simulink model "mount_2_rust"  (R2022b)
settings: Solver=FixedStepDiscrete  StartTime=0.0  StopTime=5  FixedStep=deltaT  RelTol=1e-3
InitFcn:
  | %
  | % Initialization callback function
  | %
  | 
  | try
  |    % fprintf('\n Simulink control model!\n');
  | 
  |    % Get Simulink model directory
  |    [filepath,name,ext] = fileparts(which(bdroot));
  | 
  |    if ~strcmp(filepath,pwd)
  |       fprintf('\n Changing current directory to \n %s \n',filepath);
  |       cd(filepath);
  |    end
  | 
  | catch
  |    warning('Running the InitFcn from puSimulate script');
  | end
values from neighbouring files (symbols this model uses):
  drv_delay = ceil(mount.delay/FEM_Ts)    [load_mount_data.m]
  FEM_Ts = deltaT    (= 0.000125)    [load_mount_data.m]
  Hdrive_d = c2d(o.Hdrive(1,1), FEM_Ts, 'tustin')    [load_mount_data.m]
  mnt_TF_Ts = FEM_Ts    (= 0.000125)    [load_mount_data.m]
  o = fun_confBase(oTest)    [load_mount_data.m]
undefined symbols (not defined in the file or in its folder): a, az, az_ff_en, b, c, DiscIntNeverNeededParam, el, gir, magnitude, mount
libraries: simulink x2, simulink_extras x2
(part 1 of 2)
settings Model: SimulationMode=accelerator  Creator=RRomano  LastModifiedBy=rromano
settings SolverCC: AlgebraicLoopSolver=TrustRegion
settings DataIOCC: SaveOutput=off  SignalLogging=off  DSMLogging=off  SaveTime=off  ReturnWorkspaceOutputs=off
settings OptimizationCC: DefaultParameterBehavior=Inlined  GainParamInheritBuiltInType=on  UseFloatMulNetSlope=on  UseSpecifiedMinMax=on  InlineInvariantSignals=on  StrengthReduction=on  PassReuseOutputArgsAs=Individual arguments  ZeroExternalMemoryAtStartup=off  ZeroInternalMemoryAtStartup=off  NoFixptDivByZeroProtection=on  EfficientFloat2IntCast=on  LifeSpan=1000  SimCompilerOptimization=on  AccelVerboseBuild=on  OptimizeBlockOrder=speed  OptimizationPriority=Speed  OptimizationCustomize=off  MultiThreadedLoops=on  EfficientTunableParamExpr=on
settings DebuggingCC: InheritedTsInSrcMsg=none  MultiTaskRateTransMsg=warning  ParameterTunabilityLossMsg=error  UnconnectedInputMsg=warning  UnconnectedOutputMsg=warning  UnconnectedLineMsg=warning  SFUnexpectedBacktrackingDiag=warning  SFNoUnconditionalDefaultTransitionDiag=warning  SFExecutionAtInitializationDiag=none  SFMachineParentedDataDiag=warning  ArithmeticOperatorsInVariantConditions=warning
settings HardwareCC: ProdBitPerLong=64  ProdLongLongMode=on  ProdHWDeviceType=Intel->x86-64 (Linux 64)  TargetBitPerLong=64  TargetBitPerPointer=64  TargetBitPerSizeT=64  TargetBitPerPtrDiffT=64  TargetLongLongMode=on  TargetIntDivRoundTo=Zero  TargetEndianess=LittleEndian  TargetWordSize=64  TargetHWDeviceType=MATLAB Host  ProdEqTarget=off
settings ModelReferenceCC: EnableRefExpFcnMdlSchedulingChecks=on
settings SFSimCC: SimUseLocalCustomCode=off  MATLABDynamicMemAlloc=off  CustomCodeUndefinedFunction=UseInterfaceOnly
settings RTWCC: Description=Embedded Coder  SystemTargetFile=ert.tlc  GenCodeOnly=on  GenerateMakefile=off  TemplateMakefile=ert_default_tmf  GenerateReport=on  BuildConfiguration=Faster Runs  RTWCompilerOptimization=on  CheckMdlBeforeBuild=Warning  DLArmComputeVersion=19.05
settings CodeAppCC: ForceParamTrailComments=on  IgnoreCustomStorageClasses=off  OperatorAnnotations=on  SimulinkDataObjDesc=on  SFDataObjDesc=on  InsertBlockDesc=on
settings ERTTargetCC: TargetLangStandard=C99 (ISO)  GenerateSampleERTMain=on  CombineSignalStateStructs=on  SuppressErrorStatus=on  CodeInterfacePackaging=Reusable function  SupportNonFinite=off  SupportComplex=off  InlinedParameterPlacement=NonHierarchical  RootIOFormat=Structure reference  ERTCustomFileTemplate=example_file_process.tlc
settings ConfigComp: CovMetricSettings=dw  CovSaveCumulativeToWorkspaceVar=on  CovSaveSingleToWorkspaceVar=on  CovExternalEMLEnable=off

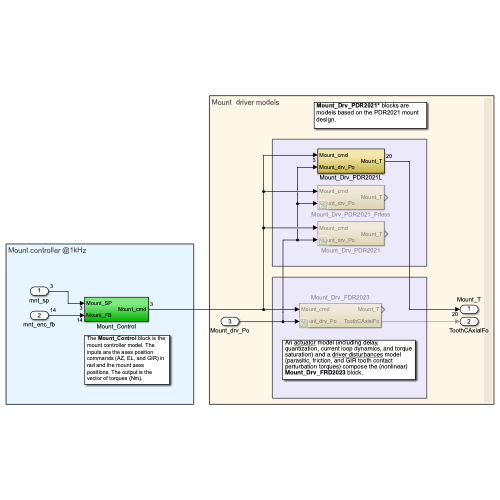
[thumbnail: Simulink's stored preview of the top-level diagram]
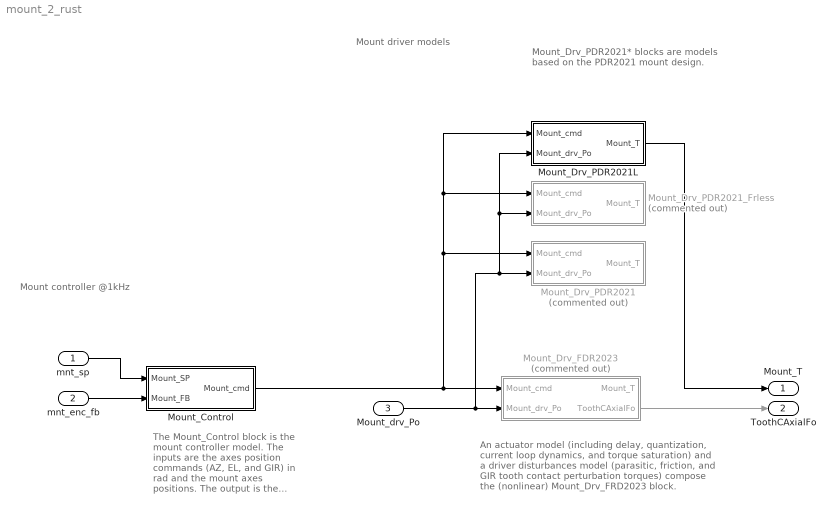
== system mount_2_rust ==
  note: Mount controller @1kHz
  note: Mount driver models
  note: The Mount_Control block is the mount controller model. The inputs are the axes position commands (AZ, EL, and GIR) in rad and the mount axes positions. The output is the vector of torques (Nm).
  note: An actuator model (including delay, quantization, current loop dynamics, and torque saturation) and a driver disturbances model (parasitic, friction, and GIR tooth contact perturbation torques) compose the (nonlinear) Mount_Drv_FRD2023 block.
  note: Mount_Drv_PDR2021* blocks are models based on the PDR2021 mount design.
  mnt_sp : Inport  SampleTime=mnt_TF_Ts
  mnt_enc_fb : Inport  Port=2  SampleTime=mnt_TF_Ts
  Mount_drv_Po : Inport  Port=3  SampleTime=FEM_Ts
  Mount_Control : Subsystem
  Mount_Drv_FDR2023 : Subsystem  Commented=on
  Mount_Drv_PDR2021 : Subsystem  Commented=on
  Mount_Drv_PDR2021L : Subsystem
  Mount_Drv_PDR2021_Frless : Subsystem  Commented=on
  Mount_T : Outport  SampleTime=FEM_Ts  VectorParamsAs1DForOutWhenUnconnected=off
  ToothCAxialFo : Outport  Port=2  SampleTime=FEM_Ts  VectorParamsAs1DForOutWhenUnconnected=off
  wires:
  mnt_sp/1 -> Mount_Control/1(Mount_SP)
  Mount_Drv_FDR2023/2(ToothCAxialFo) -> ToothCAxialFo/1
  mnt_enc_fb/1 -> Mount_Control/2(Mount_FB)
  Mount_Control/1(Mount_cmd) -> Mount_Drv_PDR2021/1(Mount_cmd), Mount_Drv_PDR2021_Frless/1(Mount_cmd), Mount_Drv_PDR2021L/1(Mount_cmd), Mount_Drv_FDR2023/1(Mount_cmd)
  Mount_drv_Po/1 -> Mount_Drv_PDR2021L/2(Mount_drv_Po), Mount_Drv_PDR2021_Frless/2(Mount_drv_Po), Mount_Drv_PDR2021/2(Mount_drv_Po), Mount_Drv_FDR2023/2(Mount_drv_Po)
  Mount_Drv_PDR2021L/1(Mount_T) -> Mount_T/1

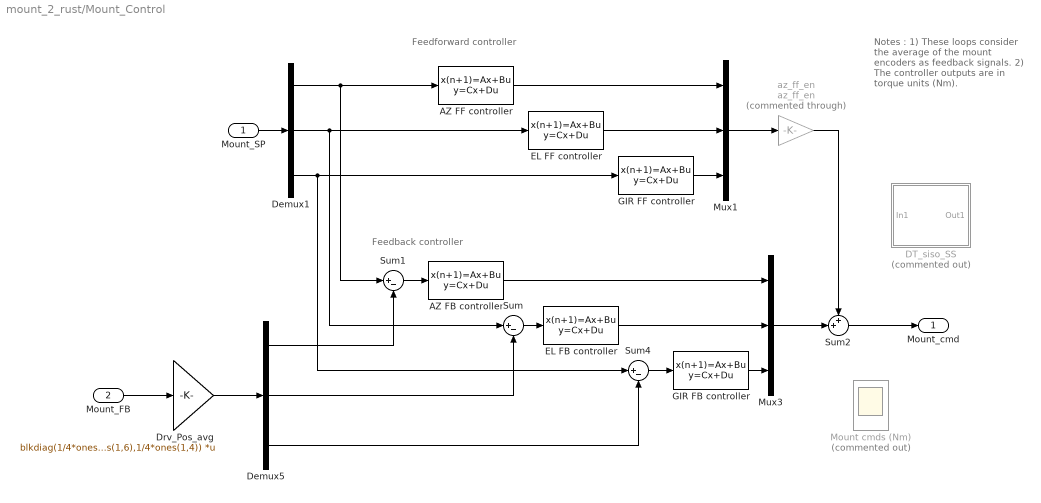
== system mount_2_rust/Mount_Control ==
  note: Feedback controller
  note: Feedforward controller
  note: Notes :
      | 1) These loops consider the average of the mount encoders as feedback signals.
      | 2) The controller outputs are in torque units (Nm).
  Mount_SP : Inport
  Mount_FB : Inport  Port=2
  AZ FB controller : DiscreteStateSpace  A=mount.az.SSdtHfb.A  B=mount.az.SSdtHfb.B  C=mount.az.SSdtHfb.C  D=mount.az.SSdtHfb.D  SampleTime=mount.az.SSdtHfb.Ts
  AZ FF controller : DiscreteStateSpace  A=mount.az.SSdtHff.A  B=mount.az.SSdtHff.B  C=mount.az.SSdtHff.C  D=mount.az.SSdtHff.D  SampleTime=mount.az.SSdtHff.Ts
  DT_siso_SS : Subsystem  Commented=on
  Demux1 : Demux  Outputs=[1,1,1]
  Demux5 : Demux  Outputs=3
  Drv_Pos_avg : Gain  Gain=blkdiag(1/4*ones(1,4),1/6*ones(1,6),1/4*ones(1,4))  Multiplication=Matrix(K*u) (u vector)
  EL FB controller : DiscreteStateSpace  A=mount.el.SSdtHfb.A  B=mount.el.SSdtHfb.B  C=mount.el.SSdtHfb.C  D=mount.el.SSdtHfb.D  SampleTime=mount.el.SSdtHfb.Ts
  EL FF controller : DiscreteStateSpace  A=mount.el.SSdtHff.A  B=mount.el.SSdtHff.B  C=mount.el.SSdtHff.C  D=mount.el.SSdtHff.D  SampleTime=mount.el.SSdtHff.Ts
  GIR FB controller : DiscreteStateSpace  A=mount.gir.SSdtHfb.A  B=mount.gir.SSdtHfb.B  C=mount.gir.SSdtHfb.C  D=mount.gir.SSdtHfb.D  SampleTime=mount.gir.SSdtHfb.Ts
  GIR FF controller : DiscreteStateSpace  A=mount.gir.SSdtHff.A  B=mount.gir.SSdtHff.B  C=mount.gir.SSdtHff.C  D=mount.gir.SSdtHff.D  SampleTime=mount.gir.SSdtHff.Ts
  Mount cmds (Nm) : Scope  Commented=on  NumInputPorts=3
  Mux1 : Mux  Inputs=[1,1,1]
  Mux3 : Mux  Inputs=[1,1,1]
  Sum : Sum  Inputs=|+-
  Sum1 : Sum  Inputs=|+-
  Sum2 : Sum  Inputs=++|
  Sum4 : Sum  Inputs=|+-
  az_ff_en : Gain  Commented=through  Gain=az_ff_en
  Mount_cmd : Outport  VectorParamsAs1DForOutWhenUnconnected=off
  wires:
  Mount_FB/1 -> Drv_Pos_avg/1
  Sum1/1 -> AZ FB controller/1
  Demux1/3 -> Sum4/1, GIR FF controller/1
  Mount_SP/1 -> Demux1/1
  Demux1/2 -> Sum/1, EL FF controller/1
  Sum/1 -> EL FB controller/1
  AZ FF controller/1 -> Mux1/1
  EL FF controller/1 -> Mux1/2
  Mux3/1 -> Sum2/2
  Sum2/1 -> Mount_cmd/1
  GIR FF controller/1 -> Mux1/3
  AZ FB controller/1 -> Mux3/1
  EL FB controller/1 -> Mux3/2
  Mux1/1 -> az_ff_en/1
  Sum4/1 -> GIR FB controller/1
  GIR FB controller/1 -> Mux3/3
  Demux5/3 -> Sum4/2
  az_ff_en/1 -> Sum2/1
  Demux1/1 -> Sum1/1, AZ FF controller/1
  Drv_Pos_avg/1 -> Demux5/1
  Demux5/2 -> Sum/2
  Demux5/1 -> Sum1/2

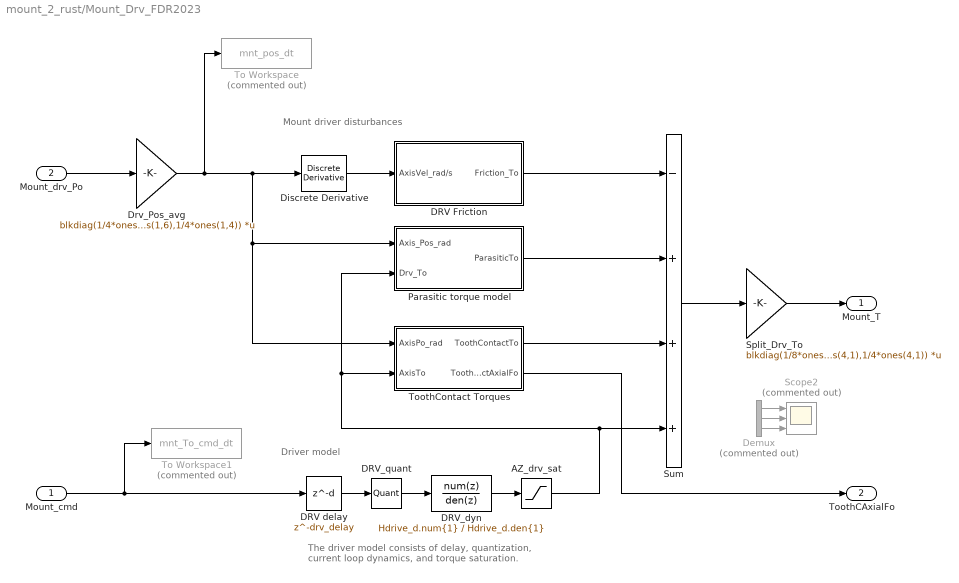
== system mount_2_rust/Mount_Drv_FDR2023 ==
  note: Driver model
  note: The driver model consists of delay, quantization, current loop dynamics, and torque saturation.
  note: Mount driver disturbances
  Mount_cmd : Inport
  Mount_drv_Po : Inport  Port=2
  AZ_drv_sat : Saturate  UpperLimit=o.vTmax  LowerLimit=-o.vTmax
  DRV Friction : Subsystem
  DRV delay : Delay  DelayLength=drv_delay  UseCircularBuffer=on  SampleTime=FEM_Ts
  DRV_dyn : DiscreteTransferFcn  Numerator=Hdrive_d.num{1}  Denominator=Hdrive_d.den{1}  SampleTime=FEM_Ts  a0EqualsOne=on
  DRV_quant : Quantizer  QuantizationInterval=o.vMotQuant_Nm
  Demux : Demux  Commented=on  Outputs=3
  Discrete Derivative : simulink/Discrete/Discrete Derivative  gainval=1  ICPrevScaledInput=0.0  OutMin=[]  OutMax=[]  OutDataType=fixdt(1, 16)  OutScaling=2^-10  DoSatur=off
  Drv_Pos_avg : Gain  Gain=blkdiag(1/4*ones(1,4),1/6*ones(1,6),1/4*ones(1,4))  Multiplication=Matrix(K*u) (u vector)
  Parasitic torque model : Subsystem
  Scope2 : Scope  Commented=on  NumInputPorts=3
  Split_Drv_To : Gain  Gain=blkdiag(1/8*ones(8,1),1/4*ones(4,1),1/4*ones(4,1))  Multiplication=Matrix(K*u) (u vector)
  Sum : Sum  Inputs=-+++
  To Workspace : ToWorkspace  Commented=on  VariableName=mnt_pos_dt  SaveFormat=Structure With Time  SampleTime=-1
  To Workspace1 : ToWorkspace  Commented=on  VariableName=mnt_To_cmd_dt  SaveFormat=Structure With Time  SampleTime=-1
  ToothContact Torques : Subsystem
  Mount_T : Outport  VectorParamsAs1DForOutWhenUnconnected=off
  ToothCAxialFo : Outport  Port=2  InitialOutput=0
  wires:
  AZ_drv_sat/1 -> Parasitic torque model/2(Drv_To), ToothContact Torques/2(AxisTo), Sum/4
  ToothContact Torques/2(ToothContactAxialFo) -> ToothCAxialFo/1
  Mount_drv_Po/1 -> Drv_Pos_avg/1
  Demux/3 -> Scope2/3
  Demux/1 -> Scope2/1
  Demux/2 -> Scope2/2
  DRV delay/1 -> DRV_quant/1
  Mount_cmd/1 -> To Workspace1/1, DRV delay/1
  DRV_quant/1 -> DRV_dyn/1
  Sum/1 -> Split_Drv_To/1
  DRV_dyn/1 -> AZ_drv_sat/1
  Drv_Pos_avg/1 -> To Workspace/1, Discrete Derivative/1, Parasitic torque model/1(Axis_Pos_rad), ToothContact Torques/1(AxisPo_rad)
  Split_Drv_To/1 -> Mount_T/1
  ToothContact Torques/1(ToothContactTo) -> Sum/3
  Parasitic torque model/1(ParasiticTo) -> Sum/2
  DRV Friction/1(Friction_To) -> Sum/1
  Discrete Derivative/1 -> DRV Friction/1(AxisVel_rad/s)

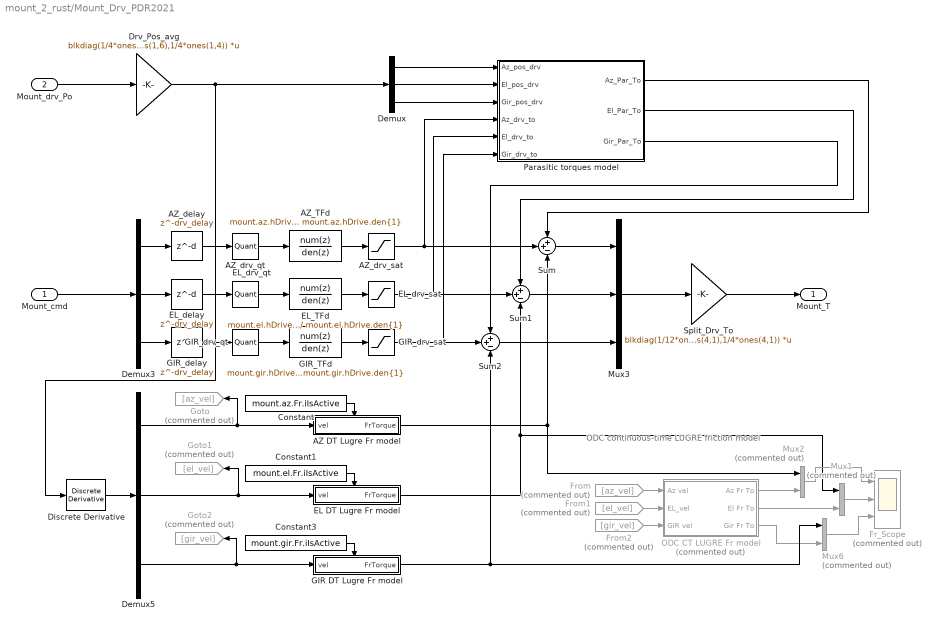
== system mount_2_rust/Mount_Drv_PDR2021 ==
  note: ODC continuous-time LUGRE friction model
  Mount_cmd : Inport
  Mount_drv_Po : Inport  Port=2
  AZ DT Lugre Fr model : Subsystem  TreatAsAtomicUnit=on  mask{frParStruct=mount.az.Fr}
      mask prompts: frParStruct "Structure with the Friction model parameters"
  AZ_TFd : DiscreteTransferFcn  Numerator=mount.az.hDrive.num{1}  Denominator=mount.az.hDrive.den{1}  SampleTime=mount.el.hDrive.Ts  a0EqualsOne=on
  AZ_delay : Delay  DelayLength=drv_delay  UseCircularBuffer=on  SampleTime=FEM_Ts
  AZ_drv_qt : Quantizer  QuantizationInterval=mount.az.driveQuant
  AZ_drv_sat : Saturate  UpperLimit=mount.az.Tmax  LowerLimit=-mount.az.Tmax
  Constant : Constant  Value=mount.az.Fr.iIsActive
  Constant1 : Constant  Value=mount.el.Fr.iIsActive
  Constant3 : Constant  Value=mount.gir.Fr.iIsActive
  Demux : Demux  Outputs=[1,1,1]
  Demux3 : Demux  Outputs=3
  Demux5 : Demux  Outputs=3%[4,6,4]
  Discrete Derivative : simulink/Discrete/Discrete Derivative  gainval=1  ICPrevScaledInput=0.0  OutMin=[]  OutMax=[]  OutDataType=fixdt(1, 16)  OutScaling=2^-10  DoSatur=off
  Drv_Pos_avg : Gain  Gain=blkdiag(1/4*ones(1,4),1/6*ones(1,6),1/4*ones(1,4))  Multiplication=Matrix(K*u) (u vector)
  EL DT Lugre Fr model : Subsystem  TreatAsAtomicUnit=on  mask{frParStruct=mount.el.Fr}
      mask prompts: frParStruct "Structure with the Friction model parameters"
  EL_TFd : DiscreteTransferFcn  Numerator=mount.el.hDrive.num{1}  Denominator=mount.el.hDrive.den{1}  SampleTime=mount.el.hDrive.Ts  a0EqualsOne=on
  EL_delay : Delay  DelayLength=drv_delay  UseCircularBuffer=on  SampleTime=FEM_Ts
  EL_drv_qt : Quantizer  QuantizationInterval=mount.el.driveQuant
  EL_drv_sat : Saturate  UpperLimit=mount.el.Tmax  LowerLimit=-mount.el.Tmax
  Fr_Scope : Scope  Commented=on  NumInputPorts=3
  From : From  Commented=on  GotoTag=az_vel
  From1 : From  Commented=on  GotoTag=el_vel
  From2 : From  Commented=on  GotoTag=gir_vel
  GIR DT Lugre Fr model : Subsystem  TreatAsAtomicUnit=on  mask{frParStruct=mount.gir.Fr}
      mask prompts: frParStruct "Structure with the Friction model parameters"
  GIR_TFd : DiscreteTransferFcn  Numerator=mount.gir.hDrive.num{1}  Denominator=mount.gir.hDrive.den{1}  SampleTime=mount.gir.hDrive.Ts  a0EqualsOne=on
  GIR_delay : Delay  DelayLength=drv_delay  UseCircularBuffer=on  SampleTime=FEM_Ts
  GIR_drv_qt : Quantizer  QuantizationInterval=mount.gir.driveQuant
  GIR_drv_sat : Saturate  UpperLimit=mount.gir.Tmax  LowerLimit=-mount.gir.Tmax
  Goto : Goto  Commented=on  GotoTag=az_vel
  Goto1 : Goto  Commented=on  GotoTag=el_vel
  Goto2 : Goto  Commented=on  GotoTag=gir_vel
  Mux1 : Mux  Commented=on  Inputs=2
  Mux2 : Mux  Commented=on  Inputs=2
  Mux3 : Mux  Inputs=3
  Mux6 : Mux  Commented=on  Inputs=2
  ODC CT LUGRE Fr model : Subsystem  Commented=on
  "Parasitic torques model " : Subsystem
  Split_Drv_To : Gain  Gain=blkdiag(1/12*ones(12,1),1/4*ones(4,1),1/4*ones(4,1))  Multiplication=Matrix(K*u) (u vector)
  Sum : Sum  Inputs=++-
  Sum1 : Sum  Inputs=++-
  Sum2 : Sum  Inputs=++-
  Mount_T : Outport  VectorParamsAs1DForOutWhenUnconnected=off
  wires:
  ODC CT LUGRE Fr model/3(Gir Fr To) -> Mux6/2
  From2/1 -> ODC CT LUGRE Fr model/3(GIR vel)
  From1/1 -> ODC CT LUGRE Fr model/2(EL_vel)
  From/1 -> ODC CT LUGRE Fr model/1(Az vel)
  Mount_cmd/1 -> Demux3/1
  ODC CT LUGRE Fr model/2(El Fr To) -> Mux1/2
  ODC CT LUGRE Fr model/1(Az Fr To) -> Mux2/2
  Demux5/2 -> EL DT Lugre Fr model/1(vel), Goto1/1
  Mux6/1 -> Fr_Scope/3
  GIR DT Lugre Fr model/1(FrTorque) -> Mux6/1, Sum2/3
  "Parasitic torques model "/3(Gir_Par_To) -> Sum2/1
  "Parasitic torques model "/2(El_Par_To) -> Sum1/1
  "Parasitic torques model "/1(Az_Par_To) -> Sum/1
  Demux5/3 -> GIR DT Lugre Fr model/1(vel), Goto2/1
  Constant1/1 -> EL DT Lugre Fr model/Enable
  Constant3/1 -> GIR DT Lugre Fr model/Enable
  GIR_drv_sat/1 -> Sum2/2, "Parasitic torques model "/6(Gir_drv_to)
  GIR_drv_qt/1 -> GIR_TFd/1
  GIR_delay/1 -> GIR_drv_qt/1
  GIR_TFd/1 -> GIR_drv_sat/1
  Demux3/3 -> GIR_delay/1
  AZ_drv_sat/1 -> Sum/2, "Parasitic torques model "/4(Az_drv_to)
  Mux1/1 -> Fr_Scope/2
  EL DT Lugre Fr model/1(FrTorque) -> Mux1/1, Sum1/3
  EL_drv_sat/1 -> Sum1/2, "Parasitic torques model "/5(El_drv_to)
  AZ DT Lugre Fr model/1(FrTorque) -> Mux2/1, Sum/3
  Mux2/1 -> Fr_Scope/1
  Constant/1 -> AZ DT Lugre Fr model/Enable
  Demux5/1 -> AZ DT Lugre Fr model/1(vel), Goto/1
  Discrete Derivative/1 -> Demux5/1
  EL_drv_qt/1 -> EL_TFd/1
  AZ_drv_qt/1 -> AZ_TFd/1
  EL_delay/1 -> EL_drv_qt/1
  AZ_delay/1 -> AZ_drv_qt/1
  Demux3/1 -> AZ_delay/1
  Demux3/2 -> EL_delay/1
  Mux3/1 -> Split_Drv_To/1
  AZ_TFd/1 -> AZ_drv_sat/1
  EL_TFd/1 -> EL_drv_sat/1
  Sum/1 -> Mux3/1
  Sum1/1 -> Mux3/2
  Sum2/1 -> Mux3/3
  Split_Drv_To/1 -> Mount_T/1
  Mount_drv_Po/1 -> Drv_Pos_avg/1
  Drv_Pos_avg/1 -> Demux/1, Discrete Derivative/1
  Demux/1 -> "Parasitic torques model "/1(Az_pos_drv)
  Demux/2 -> "Parasitic torques model "/2(El_pos_drv)
  Demux/3 -> "Parasitic torques model "/3(Gir_pos_drv)

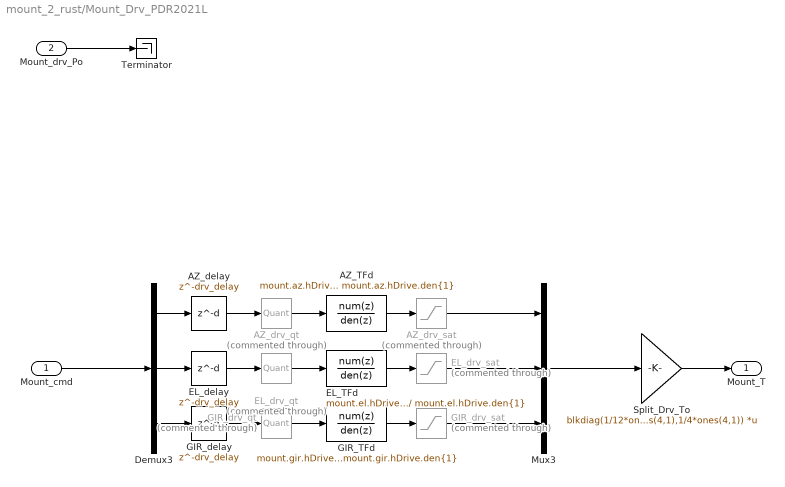
== system mount_2_rust/Mount_Drv_PDR2021L ==
  Mount_cmd : Inport
  Mount_drv_Po : Inport  Port=2
  AZ_TFd : DiscreteTransferFcn  Numerator=mount.az.hDrive.num{1}  Denominator=mount.az.hDrive.den{1}  SampleTime=mount.el.hDrive.Ts  a0EqualsOne=on
  AZ_delay : Delay  DelayLength=drv_delay  UseCircularBuffer=on  SampleTime=FEM_Ts
  AZ_drv_qt : Quantizer  Commented=through  QuantizationInterval=mount.az.driveQuant
  AZ_drv_sat : Saturate  Commented=through  UpperLimit=mount.az.Tmax  LowerLimit=-mount.az.Tmax
  Demux3 : Demux  Outputs=3
  EL_TFd : DiscreteTransferFcn  Numerator=mount.el.hDrive.num{1}  Denominator=mount.el.hDrive.den{1}  SampleTime=mount.el.hDrive.Ts  a0EqualsOne=on
  EL_delay : Delay  DelayLength=drv_delay  UseCircularBuffer=on  SampleTime=FEM_Ts
  EL_drv_qt : Quantizer  Commented=through  QuantizationInterval=mount.el.driveQuant
  EL_drv_sat : Saturate  Commented=through  UpperLimit=mount.el.Tmax  LowerLimit=-mount.el.Tmax
  GIR_TFd : DiscreteTransferFcn  Numerator=mount.gir.hDrive.num{1}  Denominator=mount.gir.hDrive.den{1}  SampleTime=mount.gir.hDrive.Ts  a0EqualsOne=on
  GIR_delay : Delay  DelayLength=drv_delay  UseCircularBuffer=on  SampleTime=FEM_Ts
  GIR_drv_qt : Quantizer  Commented=through  QuantizationInterval=mount.gir.driveQuant
  GIR_drv_sat : Saturate  Commented=through  UpperLimit=mount.gir.Tmax  LowerLimit=-mount.gir.Tmax
  Mux3 : Mux  Inputs=3%[12,4,4]
  Split_Drv_To : Gain  Gain=blkdiag(1/12*ones(12,1),1/4*ones(4,1),1/4*ones(4,1))  Multiplication=Matrix(K*u) (u vector)
  Terminator : Terminator
  Mount_T : Outport  VectorParamsAs1DForOutWhenUnconnected=off
  wires:
  Mount_cmd/1 -> Demux3/1
  GIR_drv_qt/1 -> GIR_TFd/1
  GIR_delay/1 -> GIR_drv_qt/1
  GIR_TFd/1 -> GIR_drv_sat/1
  Demux3/3 -> GIR_delay/1
  EL_drv_qt/1 -> EL_TFd/1
  AZ_drv_qt/1 -> AZ_TFd/1
  EL_delay/1 -> EL_drv_qt/1
  AZ_delay/1 -> AZ_drv_qt/1
  Demux3/1 -> AZ_delay/1
  Demux3/2 -> EL_delay/1
  Mux3/1 -> Split_Drv_To/1
  AZ_TFd/1 -> AZ_drv_sat/1
  EL_TFd/1 -> EL_drv_sat/1
  AZ_drv_sat/1 -> Mux3/1
  EL_drv_sat/1 -> Mux3/2
  GIR_drv_sat/1 -> Mux3/3
  Split_Drv_To/1 -> Mount_T/1
  Mount_drv_Po/1 -> Terminator/1

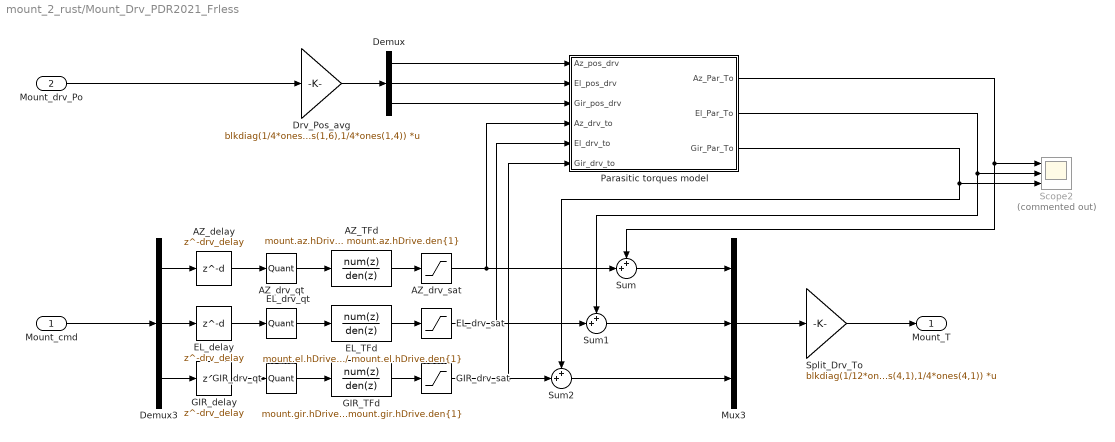
== system mount_2_rust/Mount_Drv_PDR2021_Frless ==
  Mount_cmd : Inport
  Mount_drv_Po : Inport  Port=2
  AZ_TFd : DiscreteTransferFcn  Numerator=mount.az.hDrive.num{1}  Denominator=mount.az.hDrive.den{1}  SampleTime=mount.el.hDrive.Ts  a0EqualsOne=on
  AZ_delay : Delay  DelayLength=drv_delay  UseCircularBuffer=on  SampleTime=FEM_Ts
  AZ_drv_qt : Quantizer  QuantizationInterval=mount.az.driveQuant
  AZ_drv_sat : Saturate  UpperLimit=mount.az.Tmax  LowerLimit=-mount.az.Tmax
  Demux : Demux  Outputs=[1,1,1]
  Demux3 : Demux  Outputs=3
  Drv_Pos_avg : Gain  Gain=blkdiag(1/4*ones(1,4),1/6*ones(1,6),1/4*ones(1,4))  Multiplication=Matrix(K*u) (u vector)
  EL_TFd : DiscreteTransferFcn  Numerator=mount.el.hDrive.num{1}  Denominator=mount.el.hDrive.den{1}  SampleTime=mount.el.hDrive.Ts  a0EqualsOne=on
  EL_delay : Delay  DelayLength=drv_delay  UseCircularBuffer=on  SampleTime=FEM_Ts
  EL_drv_qt : Quantizer  QuantizationInterval=mount.el.driveQuant
  EL_drv_sat : Saturate  UpperLimit=mount.el.Tmax  LowerLimit=-mount.el.Tmax
  GIR_TFd : DiscreteTransferFcn  Numerator=mount.gir.hDrive.num{1}  Denominator=mount.gir.hDrive.den{1}  SampleTime=mount.gir.hDrive.Ts  a0EqualsOne=on
  GIR_delay : Delay  DelayLength=drv_delay  UseCircularBuffer=on  SampleTime=FEM_Ts
  GIR_drv_qt : Quantizer  QuantizationInterval=mount.gir.driveQuant
  GIR_drv_sat : Saturate  UpperLimit=mount.gir.Tmax  LowerLimit=-mount.gir.Tmax
  Mux3 : Mux  Inputs=3%[12,4,4]
  "Parasitic torques model " : Subsystem
  Scope2 : Scope  Commented=on  NumInputPorts=3
  Split_Drv_To : Gain  Gain=blkdiag(1/12*ones(12,1),1/4*ones(4,1),1/4*ones(4,1))  Multiplication=Matrix(K*u) (u vector)
  Sum : Sum  Inputs=++|
  Sum1 : Sum  Inputs=++|
  Sum2 : Sum  Inputs=++|
  Mount_T : Outport  VectorParamsAs1DForOutWhenUnconnected=off
  wires:
  Mount_cmd/1 -> Demux3/1
  "Parasitic torques model "/3(Gir_Par_To) -> Scope2/3, Sum2/1
  "Parasitic torques model "/2(El_Par_To) -> Scope2/2, Sum1/1
  "Parasitic torques model "/1(Az_Par_To) -> Scope2/1, Sum/1
  GIR_drv_sat/1 -> "Parasitic torques model "/6(Gir_drv_to), Sum2/2
  GIR_drv_qt/1 -> GIR_TFd/1
  GIR_delay/1 -> GIR_drv_qt/1
  GIR_TFd/1 -> GIR_drv_sat/1
  Demux3/3 -> GIR_delay/1
  AZ_drv_sat/1 -> "Parasitic torques model "/4(Az_drv_to), Sum/2
  EL_drv_sat/1 -> "Parasitic torques model "/5(El_drv_to), Sum1/2
  EL_drv_qt/1 -> EL_TFd/1
  AZ_drv_qt/1 -> AZ_TFd/1
  EL_delay/1 -> EL_drv_qt/1
  AZ_delay/1 -> AZ_drv_qt/1
  Demux3/1 -> AZ_delay/1
  Demux3/2 -> EL_delay/1
  Mux3/1 -> Split_Drv_To/1
  AZ_TFd/1 -> AZ_drv_sat/1
  EL_TFd/1 -> EL_drv_sat/1
  Drv_Pos_avg/1 -> Demux/1
  Demux/1 -> "Parasitic torques model "/1(Az_pos_drv)
  Demux/2 -> "Parasitic torques model "/2(El_pos_drv)
  Demux/3 -> "Parasitic torques model "/3(Gir_pos_drv)
  Mount_drv_Po/1 -> Drv_Pos_avg/1
  Sum/1 -> Mux3/1
  Sum1/1 -> Mux3/2
  Sum2/1 -> Mux3/3
  Split_Drv_To/1 -> Mount_T/1

== system mount_2_rust/Mount_Control/DT_siso_SS ==
  In1 : Inport
  A : Gain  Gain=a  Multiplication=Matrix(K*u) (u vector)
  Add : Sum
  B : Gain  Gain=b
  C : Gain  Gain=c
  Unit Delay : UnitDelay  SampleTime=-1  HasFrameUpgradeWarning=on
  Out1 : Outport
  wires:
  In1/1 -> B/1
  C/1 -> Out1/1
  B/1 -> Add/1
  Add/1 -> Unit Delay/1
  A/1 -> Add/2
  Unit Delay/1 -> A/1, C/1

== system mount_2_rust/Mount_Drv_FDR2023/DRV Friction ==
  AxisVel_rad/s : Inport
  AZ DT Lugre Fr mode : Subsystem  mask{sigma0=az.oFr.sigm0, sigma1=az.oFr.sigm1, Tc=az.oFr.Tc, sigmav=az.oFr.sigmv, Ts=az.oFr.Ts, vs=az.oFr.vs, iIsSig01Active=az.oFr.iIsSig01Active}
      mask prompts: iIsSig01Active "0=inactive, 1=active"
  Constant : Constant  Value=o.az.oFr.bIsActive
  Constant1 : Constant  Value=o.el.oFr.bIsActive
  Constant3 : Constant  Value=o.gir.oFr.bIsActive
  Demux5 : Demux  Outputs=[1,1,1]
  EL DT Lugre Fr model : Subsystem  mask{sigma0=el.oFr.sigm0, sigma1=el.oFr.sigm1, Tc=el.oFr.Tc, sigmav=el.oFr.sigmv, Ts=el.oFr.Ts, vs=el.oFr.vs, iIsSig01Active=el.oFr.iIsSig01Active}
      mask prompts: iIsSig01Active "0=inactive, 1=active"
  EL DT Lugre Fr model_ : Subsystem  Commented=on  TreatAsAtomicUnit=on  mask{frParStruct=mount.el.Fr}
      mask prompts: frParStruct "Structure with the Friction model parameters"
  GIR DT Lugre Fr model : Subsystem  mask{sigma0=gir.oFr.sigm0, sigma1=gir.oFr.sigm1, Tc=gir.oFr.Tc, sigmav=gir.oFr.sigmv, Ts=gir.oFr.Ts, vs=gir.oFr.vs, iIsSig01Active=gir.oFr.iIsSig01Active}
      mask prompts: iIsSig01Active "0=inactive, 1=active"
  GIR DT Lugre Fr model_ : Subsystem  Commented=on  TreatAsAtomicUnit=on  mask{frParStruct=mount.gir.Fr}
      mask prompts: frParStruct "Structure with the Friction model parameters"
  Mux1 : Mux  Inputs=[1,1,1]
  Friction_To : Outport
  wires:
  Demux5/3 -> GIR DT Lugre Fr model/1(v)
  Demux5/2 -> EL DT Lugre Fr model/1(v)
  Demux5/1 -> AZ DT Lugre Fr mode/1(v)
  AxisVel_rad/s/1 -> Demux5/1
  Constant1/1 -> EL DT Lugre Fr model/Enable
  GIR DT Lugre Fr model/1(Tfr) -> Mux1/3
  AZ DT Lugre Fr mode/1(Tfr) -> Mux1/1
  Constant3/1 -> GIR DT Lugre Fr model/Enable
  Constant/1 -> AZ DT Lugre Fr mode/Enable
  EL DT Lugre Fr model/1(Tfr) -> Mux1/2
  Mux1/1 -> Friction_To/1

== system mount_2_rust/Mount_Drv_FDR2023/Parasitic torque model ==
  Axis_Pos_rad : Inport
  Drv_To : Inport  Port=2
  Constant1 : Constant  Value=az.oParasitic.bIsActive
  Constant2 : Constant  Value=el.oParasitic.bIsActive
  Constant3 : Constant  Value=gir.oParasitic.bIsActive
  Demux : Demux  Outputs=[1,1,1]
  Demux1 : Demux  Outputs=[1,1,1]
  Mux3 : Mux  Inputs=3
  Parasitic AZ : Subsystem  mask{oParasitic=az.oParasitic}
  Parasitic EL : Subsystem  mask{oParasitic=el.oParasitic}
  Parasitic GIR : Subsystem  mask{oParasitic=gir.oParasitic}
  Radians to Degrees : simulink_extras/Transformations/Radians to Degrees
  UnitDelay_PO : UnitDelay  Commented=through  SampleTime=-1  HasFrameUpgradeWarning=on
  UnitDelay_To : UnitDelay  Commented=through  SampleTime=-1  HasFrameUpgradeWarning=on
  ParasiticTo : Outport
  wires:
  Demux/1 -> Parasitic AZ/2(AxisPo_deg)
  Demux/2 -> Parasitic EL/2(AxisPo_deg)
  Demux/3 -> Parasitic GIR/2(AxisPo_deg)
  UnitDelay_PO/1 -> Radians to Degrees/1
  UnitDelay_To/1 -> Demux1/1
  Demux1/3 -> Parasitic GIR/1(AxisTo_Nm)
  Demux1/2 -> Parasitic EL/1(AxisTo_Nm)
  Demux1/1 -> Parasitic AZ/1(AxisTo_Nm)
  Drv_To/1 -> UnitDelay_To/1
  Constant2/1 -> Parasitic EL/Enable
  Parasitic EL/1(TotalTo) -> Mux3/2
  Radians to Degrees/1 -> Demux/1
  Constant3/1 -> Parasitic GIR/Enable
  Axis_Pos_rad/1 -> UnitDelay_PO/1
  Parasitic GIR/1(TotalTo) -> Mux3/3
  Constant1/1 -> Parasitic AZ/Enable
  Parasitic AZ/1(TotalTo) -> Mux3/1
  Mux3/1 -> ParasiticTo/1

== system mount_2_rust/Mount_Drv_FDR2023/ToothContact Torques ==
  AxisPo_rad : Inport
  AxisTo : Inport  Port=2
  Constant2 : Constant  Value=[0 0]
  Mux3 : Mux  Inputs=2
  Radians to Degrees : simulink_extras/Transformations/Radians to Degrees
  Sel : Selector  IndexMode=Zero-based  InputPortWidth=3  IndexOptions=Index vector (dialog)  Indices=[2]  OutputSizes=1
  Sel1 : Selector  IndexMode=Zero-based  InputPortWidth=3  IndexOptions=Index vector (dialog)  Indices=[2]  OutputSizes=1
  Sum1 : Sum  Inputs=|++
  ToothContact GIR (Norm) : Subsystem  mask{oToothContact=gir.oToothContactNorm}
  ToothContact GIR (Peak) : Subsystem  mask{oToothContact=gir.oToothContactPeak}
  factAxial : Gain  Gain=gir.oToothContactPeak.factAxial
  ToothContactTo : Outport
  ToothContactAxialFo : Outport  Port=2
  wires:
  ToothContact GIR (Norm)/1(TotalTo) -> Sum1/2
  Sum1/1 -> Mux3/2, factAxial/1
  Sel/1 -> Radians to Degrees/1
  Radians to Degrees/1 -> ToothContact GIR (Peak)/1(AxisPos_deg), ToothContact GIR (Norm)/1(AxisPos_deg)
  Sel1/1 -> ToothContact GIR (Peak)/2(AxisTo), ToothContact GIR (Norm)/2(AxisTo)
  Mux3/1 -> ToothContactTo/1
  AxisTo/1 -> Sel1/1
  AxisPo_rad/1 -> Sel/1
  factAxial/1 -> ToothContactAxialFo/1
  ToothContact GIR (Peak)/1(TotalTo) -> Sum1/1
  Constant2/1 -> Mux3/1

== system mount_2_rust/Mount_Drv_PDR2021/AZ DT Lugre Fr model ==
  vel : Inport
  Enable : EnablePort
  Constant : Constant  Value=frParStruct.iIsSig01Active
  Discrete-Time Integrator : DiscreteIntegrator  SampleTime=-1  ICPrevOutput=DiscIntNeverNeededParam  ICPrevScaledInput=DiscIntNeverNeededParam
  Sum : Sum  Inputs=+++
  g(v) : Subsystem
  sigma_0 : Gain  Gain=frParStruct.sigm0
  sigma_1 : Gain  Gain=frParStruct.sigm1
  sigma_v : Gain  Gain=frParStruct.sigmv
  v2z : Subsystem
  FrTorque : Outport  VectorParamsAs1DForOutWhenUnconnected=off
  wires:
  Constant/1 -> v2z/Enable, g(v)/Enable
  vel/1 -> sigma_v/1, g(v)/1(v), v2z/1(v)
  Sum/1 -> FrTorque/1
  sigma_0/1 -> Sum/2
  sigma_1/1 -> Sum/1
  v2z/1(dz) -> sigma_1/1, Discrete-Time Integrator/1
  sigma_v/1 -> Sum/3  "Viscose Friction"
  g(v)/1(g) -> v2z/2(g(v))
  Discrete-Time Integrator/1 -> v2z/3(z), sigma_0/1

== system mount_2_rust/Mount_Drv_PDR2021/EL DT Lugre Fr model ==
  vel : Inport
  Enable : EnablePort
  Constant : Constant  Value=frParStruct.iIsSig01Active
  Discrete-Time Integrator : DiscreteIntegrator  SampleTime=-1  ICPrevOutput=DiscIntNeverNeededParam  ICPrevScaledInput=DiscIntNeverNeededParam
  Sum : Sum  Inputs=+++
  To Workspace : ToWorkspace  VariableName=el_Ve  SampleTime=-1
  To Workspace1 : ToWorkspace  VariableName=el_To  SampleTime=-1
  g(v) : Subsystem
  sigma_0 : Gain  Gain=frParStruct.sigm0
  sigma_1 : Gain  Gain=frParStruct.sigm1
  sigma_v : Gain  Gain=frParStruct.sigmv
  v2z : Subsystem
  FrTorque : Outport  VectorParamsAs1DForOutWhenUnconnected=off
  wires:
  Sum/1 -> FrTorque/1, To Workspace1/1
  v2z/1(dz) -> sigma_1/1, Discrete-Time Integrator/1
  Discrete-Time Integrator/1 -> v2z/3(z), sigma_0/1
  sigma_1/1 -> Sum/1
  g(v)/1(g) -> v2z/2(g(v))
  sigma_0/1 -> Sum/2
  Constant/1 -> v2z/Enable, g(v)/Enable
  vel/1 -> sigma_v/1, To Workspace/1, g(v)/1(v), v2z/1(v)
  sigma_v/1 -> Sum/3  "Viscose Friction"

== system mount_2_rust/Mount_Drv_PDR2021/GIR DT Lugre Fr model ==
  vel : Inport
  Enable : EnablePort
  Discrete-Time Integrator : DiscreteIntegrator  SampleTime=-1  ICPrevOutput=DiscIntNeverNeededParam  ICPrevScaledInput=DiscIntNeverNeededParam
  Gain : Gain  Gain=frParStruct.iIsSig01Active
  Scope : Scope
  Sum : Sum  Inputs=+++
  To Workspace : ToWorkspace  VariableName=gir_Ve  SampleTime=-1
  To Workspace1 : ToWorkspace  VariableName=gir_To  SampleTime=-1
  g(v) : Subsystem
  sigma_0 : Gain  Gain=frParStruct.sigm0
  sigma_1 : Gain  Gain=frParStruct.sigm1
  sigma_v : Gain  Gain=frParStruct.sigmv
  v2z : Subsystem
  FrTorque : Outport  VectorParamsAs1DForOutWhenUnconnected=off
  wires:
  Gain/1 -> g(v)/1(v), v2z/1(v)
  sigma_1/1 -> Sum/1
  Sum/1 -> FrTorque/1, To Workspace1/1
  v2z/1(dz) -> sigma_1/1, Scope/1, Discrete-Time Integrator/1
  Discrete-Time Integrator/1 -> v2z/3(z), sigma_0/1
  g(v)/1(g) -> v2z/2(g(v))
  sigma_0/1 -> Sum/2
  vel/1 -> sigma_v/1, To Workspace/1, Gain/1
  sigma_v/1 -> Sum/3  "Viscose Friction"

== system mount_2_rust/Mount_Drv_PDR2021/ODC CT LUGRE Fr model ==
  Az vel : Inport
  EL_vel : Inport  Port=2
  GIR vel : Inport  Port=3
  Constant2 : Constant
  Demux1 : Demux  Outputs=3
  Friction : Subsystem
  Mux7 : Mux  Inputs=3
  Az Fr To : Outport  VectorParamsAs1DForOutWhenUnconnected=off
  El Fr To : Outport  Port=2  VectorParamsAs1DForOutWhenUnconnected=off
  Gir Fr To : Outport  Port=3  VectorParamsAs1DForOutWhenUnconnected=off
  wires:
  GIR vel/1 -> Mux7/3
  EL_vel/1 -> Mux7/2
  Az vel/1 -> Mux7/1
  Demux1/3 -> Gir Fr To/1
  Constant2/1 -> Friction/Enable
  Friction/1(FrictionTo) -> Demux1/1
  Demux1/1 -> Az Fr To/1
  Demux1/2 -> El Fr To/1
  Mux7/1 -> Friction/1(Vel)

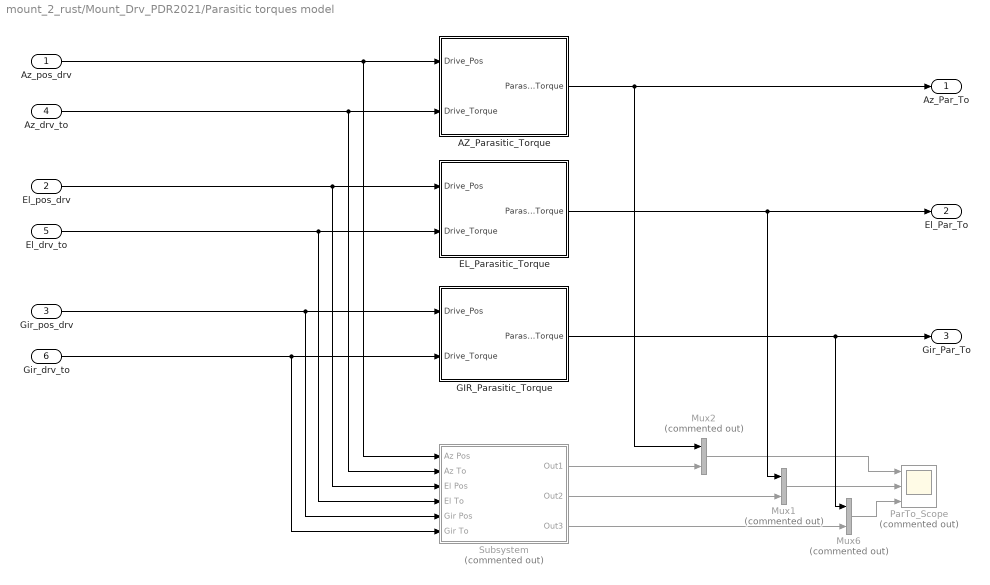
== system mount_2_rust/Mount_Drv_PDR2021/Parasitic torques model  ==
  Az_pos_drv : Inport
  El_pos_drv : Inport  Port=2
  Gir_pos_drv : Inport  Port=3
  Az_drv_to : Inport  Port=4
  El_drv_to : Inport  Port=5
  Gir_drv_to : Inport  Port=6
  AZ_Parasitic_Torque : Subsystem  mask{ParasiticModelStruc=mount.az.ParasiticTo}
      mask prompts: ParasiticModelStruc "Parasitic Torque Model Parameters Structure"
  EL_Parasitic_Torque : Subsystem  mask{ParasiticModelStruc=mount.el.ParasiticTo}
      mask prompts: ParasiticModelStruc "Parasitic Torque Model Parameters Structure"
  GIR_Parasitic_Torque : Subsystem  mask{ParasiticModelStruc=mount.gir.ParasiticTo, T_pretension=mount.gir.T_pretension}
      mask prompts: ParasiticModelStruc "Parasitic Torque Model Parameters Structure"; T_pretension "Pretension torque"
  Mux1 : Mux  Commented=on  Inputs=2
  Mux2 : Mux  Commented=on  Inputs=2
  Mux6 : Mux  Commented=on  Inputs=2
  ParTo_Scope : Scope  Commented=on  NumInputPorts=3
  Subsystem : Subsystem  Commented=on
  Az_Par_To : Outport  VectorParamsAs1DForOutWhenUnconnected=off
  El_Par_To : Outport  Port=2  VectorParamsAs1DForOutWhenUnconnected=off
  Gir_Par_To : Outport  Port=3  VectorParamsAs1DForOutWhenUnconnected=off
  wires:
  Subsystem/3(Out3) -> Mux6/2
  Subsystem/2(Out2) -> Mux1/2
  Subsystem/1(Out1) -> Mux2/2
  Mux6/1 -> ParTo_Scope/3
  Mux1/1 -> ParTo_Scope/2
  Mux2/1 -> ParTo_Scope/1
  EL_Parasitic_Torque/1(Parasitic_Torque) -> Mux1/1, El_Par_To/1
  AZ_Parasitic_Torque/1(Parasitic_Torque) -> Az_Par_To/1, Mux2/1
  El_pos_drv/1 -> EL_Parasitic_Torque/1(Drive_Pos), Subsystem/3(El Pos)
  Az_pos_drv/1 -> AZ_Parasitic_Torque/1(Drive_Pos), Subsystem/1(Az Pos)
  El_drv_to/1 -> EL_Parasitic_Torque/2(Drive_Torque), Subsystem/4(El To)
  Gir_pos_drv/1 -> GIR_Parasitic_Torque/1(Drive_Pos), Subsystem/5(Gir Pos)
  GIR_Parasitic_Torque/1(Parasitic_Torque) -> Mux6/1, Gir_Par_To/1
  Gir_drv_to/1 -> GIR_Parasitic_Torque/2(Drive_Torque), Subsystem/6(Gir To)
  Az_drv_to/1 -> AZ_Parasitic_Torque/2(Drive_Torque), Subsystem/2(Az To)

== system mount_2_rust/Mount_Drv_PDR2021_Frless/Parasitic torques model  ==
  Az_pos_drv : Inport
  El_pos_drv : Inport  Port=2
  Gir_pos_drv : Inport  Port=3
  Az_drv_to : Inport  Port=4
  El_drv_to : Inport  Port=5
  Gir_drv_to : Inport  Port=6
  AZ_Parasitic_Torque : Subsystem  mask{ParasiticModelStruc=mount.az.ParasiticTo}
      mask prompts: ParasiticModelStruc "Parasitic Torque Model Parameters Structure"
  EL_Parasitic_Torque : Subsystem  mask{ParasiticModelStruc=mount.el.ParasiticTo}
      mask prompts: ParasiticModelStruc "Parasitic Torque Model Parameters Structure"
  GIR_Parasitic_Torque : Subsystem  mask{ParasiticModelStruc=mount.gir.ParasiticTo, T_pretension=mount.gir.T_pretension}
      mask prompts: ParasiticModelStruc "Parasitic Torque Model Parameters Structure"; T_pretension "Pretension torque"
  Mux1 : Mux  Commented=on  Inputs=2
  Mux2 : Mux  Commented=on  Inputs=2
  Mux6 : Mux  Commented=on  Inputs=2
  ParTo_Scope : Scope  Commented=on  NumInputPorts=3
  Subsystem : Subsystem  Commented=on
  Az_Par_To : Outport  VectorParamsAs1DForOutWhenUnconnected=off
  El_Par_To : Outport  Port=2  VectorParamsAs1DForOutWhenUnconnected=off
  Gir_Par_To : Outport  Port=3  VectorParamsAs1DForOutWhenUnconnected=off
  wires:
  Subsystem/3(Out3) -> Mux6/2
  Subsystem/2(Out2) -> Mux1/2
  Subsystem/1(Out1) -> Mux2/2
  Mux6/1 -> ParTo_Scope/3
  Mux1/1 -> ParTo_Scope/2
  Mux2/1 -> ParTo_Scope/1
  EL_Parasitic_Torque/1(Parasitic_Torque) -> Mux1/1, El_Par_To/1
  AZ_Parasitic_Torque/1(Parasitic_Torque) -> Az_Par_To/1, Mux2/1
  El_pos_drv/1 -> EL_Parasitic_Torque/1(Drive_Pos), Subsystem/3(El Pos)
  Az_pos_drv/1 -> AZ_Parasitic_Torque/1(Drive_Pos), Subsystem/1(Az Pos)
  El_drv_to/1 -> EL_Parasitic_Torque/2(Drive_Torque), Subsystem/4(El To)
  Gir_pos_drv/1 -> GIR_Parasitic_Torque/1(Drive_Pos), Subsystem/5(Gir Pos)
  GIR_Parasitic_Torque/1(Parasitic_Torque) -> Mux6/1, Gir_Par_To/1
  Gir_drv_to/1 -> GIR_Parasitic_Torque/2(Drive_Torque), Subsystem/6(Gir To)
  Az_drv_to/1 -> AZ_Parasitic_Torque/2(Drive_Torque), Subsystem/2(Az To)

== system mount_2_rust/Mount_Drv_FDR2023/DRV Friction/AZ DT Lugre Fr mode ==
  v : Inport
  Enable : EnablePort
  Constant : Constant  Value=iIsSig01Active
  Discrete-Time Integrator : DiscreteIntegrator  SampleTime=-1  ICPrevOutput=DiscIntNeverNeededParam  ICPrevScaledInput=DiscIntNeverNeededParam
  Sum : Sum  Inputs=+++
  g(v) : Subsystem
  sigma_0 : Gain  Gain=sigma0
  sigma_1 : Gain  Gain=sigma1
  sigma_v : Gain  Gain=sigmav
  v2z : Subsystem
  Tfr : Outport
  wires:
  Constant/1 -> g(v)/Enable, v2z/Enable
  v/1 -> sigma_v/1, v2z/1(v), g(v)/1(v)
  sigma_v/1 -> Sum/3
  sigma_1/1 -> Sum/1
  Sum/1 -> Tfr/1
  sigma_0/1 -> Sum/2
  g(v)/1(g) -> v2z/2(g(v))
  Discrete-Time Integrator/1 -> v2z/3(z), sigma_0/1
  v2z/1(dz) -> sigma_1/1, Discrete-Time Integrator/1

== system mount_2_rust/Mount_Drv_FDR2023/DRV Friction/EL DT Lugre Fr model ==
  v : Inport
  Enable : EnablePort
  Constant : Constant  Value=iIsSig01Active
  Discrete-Time Integrator : DiscreteIntegrator  SampleTime=-1  ICPrevOutput=DiscIntNeverNeededParam  ICPrevScaledInput=DiscIntNeverNeededParam
  Sum : Sum  Inputs=+++
  g(v) : Subsystem
  sigma_0 : Gain  Gain=sigma0
  sigma_1 : Gain  Gain=sigma1
  sigma_v : Gain  Gain=sigmav
  v2z : Subsystem
  Tfr : Outport
  wires:
  Constant/1 -> g(v)/Enable, v2z/Enable
  sigma_0/1 -> Sum/2
  Discrete-Time Integrator/1 -> v2z/3(z), sigma_0/1
  g(v)/1(g) -> v2z/2(g(v))
  v/1 -> sigma_v/1, v2z/1(v), g(v)/1(v)
  Sum/1 -> Tfr/1
  sigma_1/1 -> Sum/1
  v2z/1(dz) -> sigma_1/1, Discrete-Time Integrator/1
  sigma_v/1 -> Sum/3

== system mount_2_rust/Mount_Drv_FDR2023/DRV Friction/EL DT Lugre Fr model_ ==
  vel : Inport
  Enable : EnablePort
  Constant : Constant  Value=frParStruct.iIsSig01Active
  Discrete-Time Integrator : DiscreteIntegrator  SampleTime=-1  ICPrevOutput=DiscIntNeverNeededParam  ICPrevScaledInput=DiscIntNeverNeededParam
  Sum : Sum  Inputs=+++
  To Workspace : ToWorkspace  VariableName=el_Ve  SampleTime=-1
  To Workspace1 : ToWorkspace  VariableName=el_To  SampleTime=-1
  g(v) : Subsystem
  sigma_0 : Gain  Gain=frParStruct.sigm0
  sigma_1 : Gain  Gain=frParStruct.sigm1
  sigma_v : Gain  Gain=frParStruct.sigmv
  v2z : Subsystem
  FrTorque : Outport  VectorParamsAs1DForOutWhenUnconnected=off
  wires:
  Sum/1 -> FrTorque/1, To Workspace1/1
  v2z/1(dz) -> sigma_1/1, Discrete-Time Integrator/1
  Discrete-Time Integrator/1 -> v2z/3(z), sigma_0/1
  sigma_1/1 -> Sum/1
  g(v)/1(g) -> v2z/2(g(v))
  sigma_0/1 -> Sum/2
  Constant/1 -> v2z/Enable, g(v)/Enable
  vel/1 -> sigma_v/1, To Workspace/1, g(v)/1(v), v2z/1(v)
  sigma_v/1 -> Sum/3  "Viscose Friction"

== system mount_2_rust/Mount_Drv_FDR2023/DRV Friction/GIR DT Lugre Fr model ==
  note: Discretized blocks
  v : Inport
  Enable : EnablePort
  Discrete Transfer Fcn : DiscreteTransferFcn  Numerator=[1 1]  Denominator="[1+(1/pi/20/FEM_Ts),  (1-(1/pi/20/FEM_Ts))]"  SampleTime=FEM_Ts
  Discrete-Time Integrator : DiscreteIntegrator  SampleTime=FEM_Ts  ICPrevOutput=DiscIntNeverNeededParam  ICPrevScaledInput=DiscIntNeverNeededParam
  Sum : Sum  Inputs=+++
  g(v) : Subsystem
  iIsSig01Active : Gain  Gain=iIsSig01Active
  on/off : Gain  Commented=through
  sigma_0 : Gain  Gain=sigma0
  sigma_1 : Gain  Gain=sigma1
  sigma_v : Gain  Gain=sigmav
  v2z : Subsystem
      settings: MinAlgLoopOccurrences=on
  Tfr : Outport
  wires:
  Discrete Transfer Fcn/1 -> sigma_1/1
  on/off/1 -> Sum/1
  sigma_1/1 -> on/off/1
  Sum/1 -> Tfr/1
  v/1 -> sigma_v/1, iIsSig01Active/1
  iIsSig01Active/1 -> v2z/1(v), g(v)/1(v)
  sigma_v/1 -> Sum/3
  sigma_0/1 -> Sum/2
  Discrete-Time Integrator/1 -> v2z/3(z), sigma_0/1
  v2z/1(dz) -> Discrete Transfer Fcn/1, Discrete-Time Integrator/1
  g(v)/1(g) -> v2z/2(g(v))

== system mount_2_rust/Mount_Drv_FDR2023/DRV Friction/GIR DT Lugre Fr model_ ==
  vel : Inport
  Enable : EnablePort
  Discrete-Time Integrator : DiscreteIntegrator  SampleTime=-1  ICPrevOutput=DiscIntNeverNeededParam  ICPrevScaledInput=DiscIntNeverNeededParam
  Gain : Gain  Gain=frParStruct.iIsSig01Active
  Scope : Scope  Commented=on  NumInputPorts=2
  Scope1 : Scope  NumInputPorts=3
  Sum : Sum  Inputs=+++
  To Workspace : ToWorkspace  VariableName=gir_Ve  SampleTime=-1
  To Workspace1 : ToWorkspace  VariableName=gir_To  SampleTime=-1
  g(v) : Subsystem
  sigma_0 : Gain  Gain=frParStruct.sigm0
  sigma_1 : Gain  Gain=frParStruct.sigm1
  sigma_v : Gain  Gain=frParStruct.sigmv
  v2z : Subsystem
  FrTorque : Outport  VectorParamsAs1DForOutWhenUnconnected=off
  wires:
  sigma_1/1 -> Sum/1, Scope1/1  "sigma1*dz"
  sigma_0/1 -> Sum/2, Scope1/2  "sigma0*z"
  Gain/1 -> g(v)/1(v), v2z/1(v)
  Sum/1 -> FrTorque/1, To Workspace1/1
  v2z/1(dz) -> Scope/1, sigma_1/1, Discrete-Time Integrator/1  "dz"
  Discrete-Time Integrator/1 -> v2z/3(z), sigma_0/1, Scope/2  "z"
  g(v)/1(g) -> v2z/2(g(v))
  vel/1 -> sigma_v/1, To Workspace/1, Gain/1
  sigma_v/1 -> Sum/3, Scope1/3  "Viscous Friction"

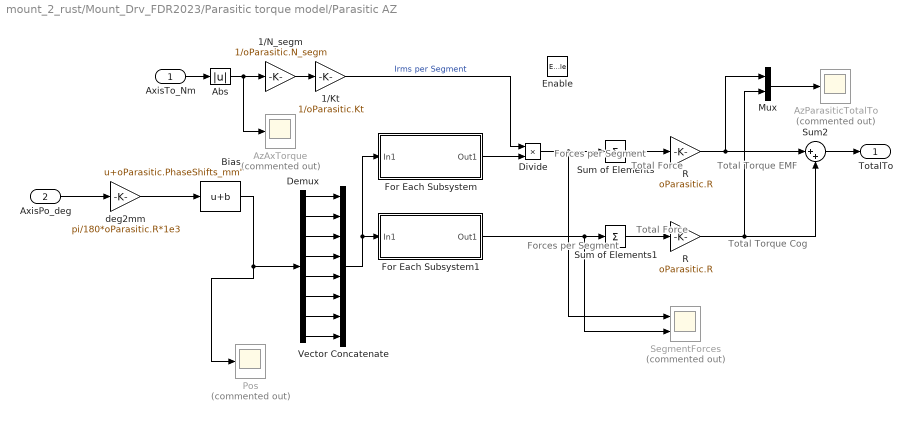
== system mount_2_rust/Mount_Drv_FDR2023/Parasitic torque model/Parasitic AZ ==
  note: Total
      | Torque Cog
  note: Total
      | Torque EMF
  note: Total
      | Force
  note: Forces per
      | Segment
  note: Forces per
      | Segment
  note: Total
      | Force
  AxisTo_Nm : Inport
  AxisPo_deg : Inport  Port=2
  Enable : EnablePort
  1/Kt : Gain  Gain=1/oParasitic.Kt
  1/N_segm : Gain  Gain=1/oParasitic.N_segm
  Abs : Abs  SaturateOnIntegerOverflow=off
  AzAxTorque : Scope  Commented=on
  AzParasiticTotalTo : Scope  Commented=on
  Bias : Bias  Bias=oParasitic.PhaseShifts_mm'  SaturateOnIntegerOverflow=off
  Demux : Demux  Outputs=8
  Divide : Product  Inputs=**
  For Each Subsystem : Subsystem  TreatAsAtomicUnit=on
  For Each Subsystem1 : Subsystem  TreatAsAtomicUnit=on
  Mux : Mux  Inputs=2
  Pos : Scope  Commented=on
  R : Gain  Gain=oParasitic.R
  "R " : Gain  Gain=oParasitic.R
  SegmentForces : Scope  Commented=on  NumInputPorts=2
  Sum of Elements : Sum  Inputs=+
  Sum of Elements1 : Sum  Inputs=+
  Sum2 : Sum  Inputs=|++
  Vector Concatenate : Concatenate  NumInputs=oParasitic.N_segm
  deg2mm : Gain  Gain=pi/180*oParasitic.R*1e3
  TotalTo : Outport
  wires:
  AxisPo_deg/1 -> deg2mm/1
  deg2mm/1 -> Bias/1
  Abs/1 -> 1/N_segm/1, AzAxTorque/1
  AxisTo_Nm/1 -> Abs/1
  Demux/8 -> Vector Concatenate/8
  Demux/7 -> Vector Concatenate/7
  Demux/6 -> Vector Concatenate/6
  Demux/5 -> Vector Concatenate/5
  Demux/4 -> Vector Concatenate/4
  Demux/3 -> Vector Concatenate/3
  Demux/2 -> Vector Concatenate/2
  Demux/1 -> Vector Concatenate/1
  For Each Subsystem1/1(Out1) -> Sum of Elements1/1, SegmentForces/2
  For Each Subsystem/1(Out1) -> Divide/2
  Vector Concatenate/1 -> For Each Subsystem1/1(In1), For Each Subsystem/1(In1)
  Bias/1 -> Pos/1, Demux/1
  Mux/1 -> AzParasiticTotalTo/1
  1/Kt/1 -> Divide/1  "Irms per Segment"
  Sum of Elements/1 -> R/1
  1/N_segm/1 -> 1/Kt/1
  R/1 -> Sum2/1, Mux/1
  "R "/1 -> Mux/2, Sum2/2
  Divide/1 -> SegmentForces/1, Sum of Elements/1
  Sum2/1 -> TotalTo/1
  Sum of Elements1/1 -> "R "/1

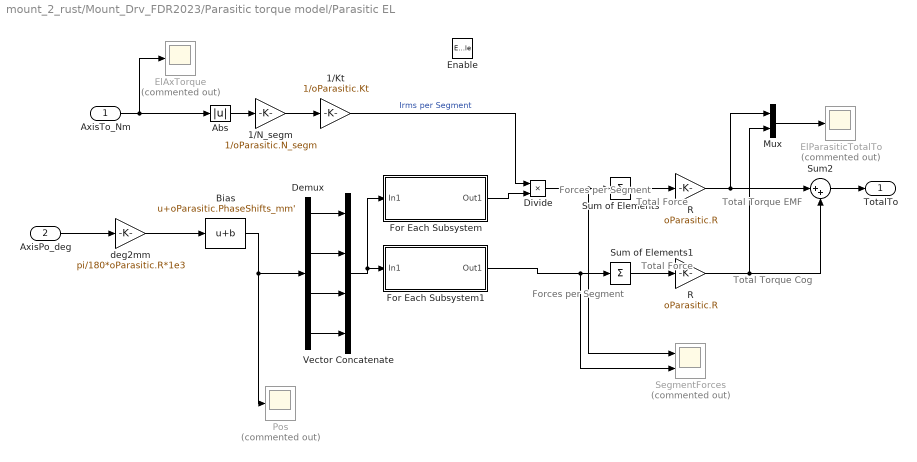
== system mount_2_rust/Mount_Drv_FDR2023/Parasitic torque model/Parasitic EL ==
  note: Total
      | Torque Cog
  note: Total
      | Torque EMF
  note: Total
      | Force
  note: Forces per
      | Segment
  note: Forces per
      | Segment
  note: Total
      | Force
  AxisTo_Nm : Inport
  AxisPo_deg : Inport  Port=2
  Enable : EnablePort
  1/Kt : Gain  Gain=1/oParasitic.Kt
  1/N_segm : Gain  Gain=1/oParasitic.N_segm
  Abs : Abs  SaturateOnIntegerOverflow=off
  Bias : Bias  Bias=oParasitic.PhaseShifts_mm'  SaturateOnIntegerOverflow=off
  Demux : Demux  Outputs=oParasitic.N_segm
  Divide : Product  Inputs=**
  ElAxTorque : Scope  Commented=on
  ElParasiticTotalTo : Scope  Commented=on
  For Each Subsystem : Subsystem  TreatAsAtomicUnit=on
  For Each Subsystem1 : Subsystem  TreatAsAtomicUnit=on
  Mux : Mux  Inputs=2
  Pos : Scope  Commented=on
  R : Gain  Gain=oParasitic.R
  "R " : Gain  Gain=oParasitic.R
  SegmentForces : Scope  Commented=on  NumInputPorts=2
  Sum of Elements : Sum  Inputs=+
  Sum of Elements1 : Sum  Inputs=+
  Sum2 : Sum  Inputs=|++
  Vector Concatenate : Concatenate  NumInputs=oParasitic.N_segm
  deg2mm : Gain  Gain=pi/180*oParasitic.R*1e3
  TotalTo : Outport
  wires:
  AxisPo_deg/1 -> deg2mm/1
  deg2mm/1 -> Bias/1
  Abs/1 -> 1/N_segm/1
  AxisTo_Nm/1 -> Abs/1, ElAxTorque/1
  Demux/4 -> Vector Concatenate/4
  Demux/3 -> Vector Concatenate/3
  Demux/2 -> Vector Concatenate/2
  Demux/1 -> Vector Concatenate/1
  For Each Subsystem1/1(Out1) -> Sum of Elements1/1, SegmentForces/2
  For Each Subsystem/1(Out1) -> Divide/2
  Vector Concatenate/1 -> For Each Subsystem1/1(In1), For Each Subsystem/1(In1)
  Bias/1 -> Demux/1, Pos/1
  Mux/1 -> ElParasiticTotalTo/1
  1/Kt/1 -> Divide/1  "Irms per Segment"
  Sum of Elements/1 -> R/1
  1/N_segm/1 -> 1/Kt/1
  R/1 -> Sum2/1, Mux/1
  "R "/1 -> Mux/2, Sum2/2
  Divide/1 -> SegmentForces/1, Sum of Elements/1
  Sum2/1 -> TotalTo/1
  Sum of Elements1/1 -> "R "/1

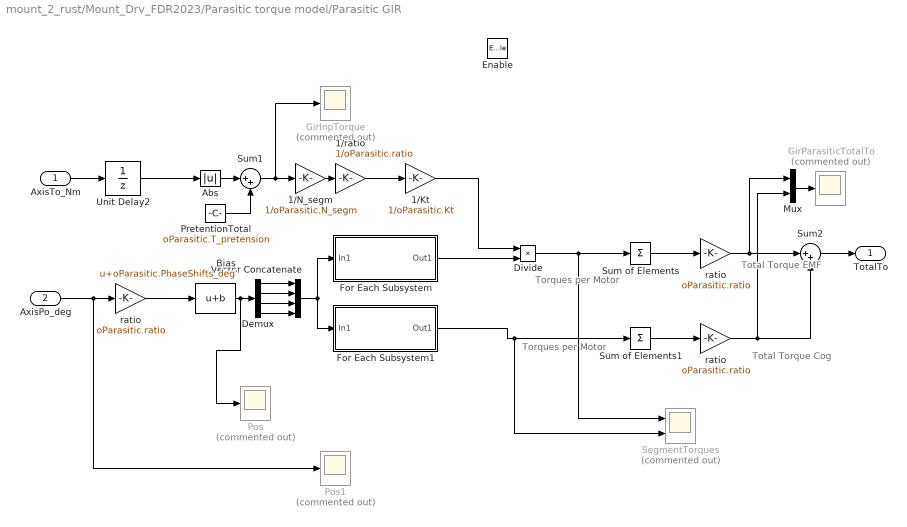
== system mount_2_rust/Mount_Drv_FDR2023/Parasitic torque model/Parasitic GIR ==
  note: Total
      | Torque Cog
  note: Total
      | Torque EMF
  note: Torques
      | per Motor
  note: Torques per
      | Motor
  AxisTo_Nm : Inport
  AxisPo_deg : Inport  Port=2
  Enable : EnablePort
  1/Kt : Gain  Gain=1/oParasitic.Kt
  1/N_segm : Gain  Gain=1/oParasitic.N_segm
  "1/ratio   " : Gain  Gain=1/oParasitic.ratio
  Abs : Abs  SaturateOnIntegerOverflow=off
  Bias : Bias  Bias=oParasitic.PhaseShifts_deg'  SaturateOnIntegerOverflow=off
  Demux : Demux
  Divide : Product  Inputs=**
  For Each Subsystem : Subsystem  TreatAsAtomicUnit=on
  For Each Subsystem1 : Subsystem  TreatAsAtomicUnit=on
  GirInpTorque : Scope  Commented=on
  GirParasiticTotalTo : Scope  Commented=on
  Mux : Mux  Inputs=2
  Pos : Scope  Commented=on
  Pos1 : Scope  Commented=on
  PretentionTotal : Constant  Value=oParasitic.T_pretension
  SegmentTorques : Scope  Commented=on  NumInputPorts=2
  Sum of Elements : Sum  Inputs=+
  Sum of Elements1 : Sum  Inputs=+
  Sum1 : Sum  Inputs=|++
  Sum2 : Sum  Inputs=|++
  Unit Delay2 : UnitDelay  SampleTime=-1  HasFrameUpgradeWarning=on
  Vector Concatenate : Concatenate  NumInputs=oParasitic.N_segm
  ratio : Gain  Gain=oParasitic.ratio
  "ratio " : Gain  Gain=oParasitic.ratio
  "ratio  " : Gain  Gain=oParasitic.ratio
  TotalTo : Outport
  wires:
  Unit Delay2/1 -> Abs/1
  AxisTo_Nm/1 -> Unit Delay2/1
  Sum1/1 -> 1/N_segm/1, GirInpTorque/1
  1/Kt/1 -> Divide/1
  PretentionTotal/1 -> Sum1/2
  Abs/1 -> Sum1/1
  "1/ratio   "/1 -> 1/Kt/1
  1/N_segm/1 -> "1/ratio   "/1
  Bias/1 -> Demux/1, Pos/1
  Demux/4 -> Vector Concatenate/4
  Demux/3 -> Vector Concatenate/3
  Demux/2 -> Vector Concatenate/2
  Demux/1 -> Vector Concatenate/1
  Vector Concatenate/1 -> For Each Subsystem1/1(In1), For Each Subsystem/1(In1)
  For Each Subsystem/1(Out1) -> Divide/2
  For Each Subsystem1/1(Out1) -> Sum of Elements1/1, SegmentTorques/2
  "ratio  "/1 -> Sum2/1, Mux/1
  "ratio "/1 -> Mux/2, Sum2/2
  Sum of Elements/1 -> "ratio  "/1
  Sum of Elements1/1 -> "ratio "/1
  ratio/1 -> Bias/1
  AxisPo_deg/1 -> ratio/1, Pos1/1
  Mux/1 -> GirParasiticTotalTo/1
  Divide/1 -> Sum of Elements/1, SegmentTorques/1
  Sum2/1 -> TotalTo/1

== system mount_2_rust/Mount_Drv_FDR2023/ToothContact Torques/ToothContact GIR (Norm) ==
  AxisPos_deg : Inport
  AxisTo : Inport  Port=2
  1-D Lookup Table : Lookup_n-D  NumberOfTableDimensions=1  BreakpointsForDimension1=oToothContact.oInterp.Pos  Table=oToothContact.oInterp.TorqueRate  InternalRulePriority=Speed  RndMeth=Simplest
  Abs : Abs  SaturateOnIntegerOverflow=off
  Gain : Gain  Gain=0.25
  Max Position : Constant  Value=oToothContact.maxPos
  Phase Shifts : Constant  Value=oToothContact.PhaseShift_deg
  PretensionTotal : Constant  Value=gir.T_pretension
  Product1 : Product  RndMeth=Zero
  Rem : Math  Operator=rem
  Sum of Elements : Sum  Inputs=+  CollapseMode=Specified dimension
  Sum1 : Sum  Inputs=|++
  Sum2 : Sum  Inputs=|++
  TotalTo : Outport
  wires:
  AxisTo/1 -> Abs/1
  Gain/1 -> Product1/2
  Sum1/1 -> Gain/1
  PretensionTotal/1 -> Sum1/2
  Abs/1 -> Sum1/1
  AxisPos_deg/1 -> Sum2/1
  Sum of Elements/1 -> TotalTo/1
  Phase Shifts/1 -> Sum2/2
  Sum2/1 -> Rem/1
  1-D Lookup Table/1 -> Product1/1
  Rem/1 -> 1-D Lookup Table/1
  Max Position/1 -> Rem/2
  Product1/1 -> Sum of Elements/1  "Position"

== system mount_2_rust/Mount_Drv_FDR2023/ToothContact Torques/ToothContact GIR (Peak) ==
  AxisPos_deg : Inport
  AxisTo : Inport  Port=2
  1-D Lookup Table : Lookup_n-D  NumberOfTableDimensions=1  BreakpointsForDimension1=oToothContact.oInterp.Pos  Table=oToothContact.oInterp.TorqueRate  InternalRulePriority=Speed  RndMeth=Simplest
  Abs : Abs  SaturateOnIntegerOverflow=off
  Gain : Gain  Gain=0.25
  Max Position : Constant  Value=oToothContact.maxPos
  Phase Shifts : Constant  Value=oToothContact.PhaseShift_deg
  PretensionTotal : Constant  Value=gir.T_pretension
  Product1 : Product  RndMeth=Zero
  Rem : Math  Operator=rem
  Sum of Elements : Sum  Inputs=+  CollapseMode=Specified dimension
  Sum1 : Sum  Inputs=|++
  Sum2 : Sum  Inputs=|++
  TotalTo : Outport
  wires:
  AxisTo/1 -> Abs/1
  Gain/1 -> Product1/2
  Sum1/1 -> Gain/1
  PretensionTotal/1 -> Sum1/2
  Abs/1 -> Sum1/1
  AxisPos_deg/1 -> Sum2/1
  Sum of Elements/1 -> TotalTo/1
  Phase Shifts/1 -> Sum2/2
  Sum2/1 -> Rem/1
  1-D Lookup Table/1 -> Product1/1
  Rem/1 -> 1-D Lookup Table/1
  Max Position/1 -> Rem/2
  Product1/1 -> Sum of Elements/1  "Position"

== system mount_2_rust/Mount_Drv_PDR2021/AZ DT Lugre Fr model/g(v) ==
  v : Inport
  Enable : EnablePort
  Constant : Constant  Value=0
  gs : Subsystem
  g : Outport  VectorParamsAs1DForOutWhenUnconnected=off
  wires:
  Constant/1 -> gs/Enable
  v/1 -> gs/1(v)
  gs/1(gs(v)) -> g/1

== system mount_2_rust/Mount_Drv_PDR2021/AZ DT Lugre Fr model/v2z ==
  v : Inport
  g(v) : Inport  Port=2
  z : Inport  Port=3
  Enable : EnablePort
  Abs : Abs  SaturateOnIntegerOverflow=off
  Divide : Product  Inputs=*/*
  Sum : Sum  Inputs=|+-
  dz : Outport  VectorParamsAs1DForOutWhenUnconnected=off
  wires:
  z/1 -> Divide/3
  g(v)/1 -> Divide/2
  Sum/1 -> dz/1
  v/1 -> Abs/1, Sum/1
  Divide/1 -> Sum/2
  Abs/1 -> Divide/1

== system mount_2_rust/Mount_Drv_PDR2021/EL DT Lugre Fr model/g(v) ==
  v : Inport
  Enable : EnablePort
  Constant : Constant  Value=0
  Sum : Sum  Inputs=|++
  gc : Constant  Value=frParStruct.Tc/frParStruct.sigm0
  gs : Subsystem
  g : Outport  VectorParamsAs1DForOutWhenUnconnected=off
  wires:
  gc/1 -> Sum/2
  Constant/1 -> gs/Enable
  gs/1(gs(v)) -> Sum/1
  v/1 -> gs/1(v)
  Sum/1 -> g/1

== system mount_2_rust/Mount_Drv_PDR2021/EL DT Lugre Fr model/v2z ==
  v : Inport
  g(v) : Inport  Port=2
  z : Inport  Port=3
  Enable : EnablePort
  Abs : Abs  SaturateOnIntegerOverflow=off
  Divide : Product  Inputs=*/*
  Sum : Sum  Inputs=|+-
  dz : Outport  VectorParamsAs1DForOutWhenUnconnected=off
  wires:
  z/1 -> Divide/3
  g(v)/1 -> Divide/2
  Sum/1 -> dz/1
  v/1 -> Abs/1, Sum/1
  Divide/1 -> Sum/2
  Abs/1 -> Divide/1

== system mount_2_rust/Mount_Drv_PDR2021/GIR DT Lugre Fr model/g(v) ==
  v : Inport
  Constant : Constant  Value=0
  Sum : Sum  Inputs=|++
  gc : Constant  Value=frParStruct.Tc/frParStruct.sigm0
  gs : Subsystem
  g : Outport  VectorParamsAs1DForOutWhenUnconnected=off
  wires:
  Constant/1 -> gs/Enable
  gc/1 -> Sum/2
  gs/1(gs(v)) -> Sum/1
  v/1 -> gs/1(v)
  Sum/1 -> g/1

== system mount_2_rust/Mount_Drv_PDR2021/GIR DT Lugre Fr model/v2z ==
  v : Inport
  g(v) : Inport  Port=2
  z : Inport  Port=3
  Abs : Abs  SaturateOnIntegerOverflow=off
  Divide : Product  Inputs=*/*
  Sum : Sum  Inputs=|+-
  dz : Outport  VectorParamsAs1DForOutWhenUnconnected=off
  wires:
  z/1 -> Divide/3
  g(v)/1 -> Divide/2
  Sum/1 -> dz/1
  v/1 -> Abs/1, Sum/1
  Divide/1 -> Sum/2
  Abs/1 -> Divide/1
